simulink model "target_generation_test"  (R2016b)
settings: Solver=VariableStepAuto  StartTime=0.0  StopTime=1  RelTol=1e-3
values from neighbouring files (symbols this model uses):
  fsw_params = init_fsw_params()    [target_generation_test_init.m]
  sc2gs_eci_unit = [-0.2821; 0.7163; 0.6382]    [target_generation_test_init.m]
  sc2sun_eci_unit = zeros(3,1)    [target_generation_test_init.m]
  sc_mode = 31    [target_generation_test_init.m]
  sc_quat = [1; 0; 0; 0]    [target_generation_test_init.m]
  vel_eci_kmps = [0.9082; 0.3185; 0.2715]    [target_generation_test_init.m]
libraries: aerolibtransform2 x1, target_generation_lib x1
settings Model: Creator=Taylor  LastModifiedBy=taylorreynolds

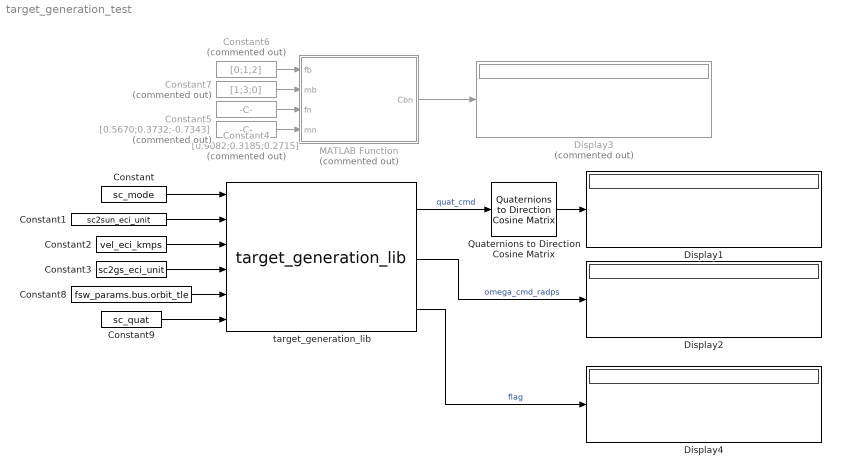
== system target_generation_test ==
  Constant : Constant  Value=sc_mode
  Constant1 : Constant  Value=sc2sun_eci_unit
  Constant2 : Constant  Value=vel_eci_kmps
  Constant3 : Constant  Value=sc2gs_eci_unit
  Constant4 : Constant  Commented=on  Value=[0.9082;0.3185;0.2715]
  Constant5 : Constant  Commented=on  Value=[0.5670;0.3732;-0.7343]
  Constant6 : Constant  Commented=on  Value=[0;1;2]
  Constant7 : Constant  Commented=on  Value=[1;3;0]
  Constant8 : Constant  Value=fsw_params.bus.orbit_tle
  Constant9 : Constant  Value=sc_quat
  Display1 : Display
  Display2 : Display
  Display3 : Display  Commented=on
  Display4 : Display
  MATLAB Function : MATLAB Function  Commented=on  TreatAsAtomicUnit=on
  Quaternions to Direction Cosine Matrix : aerolibtransform2/Quaternions to  Direction Cosine Matrix
  target_generation_lib : target_generation_lib/target_generation_lib
  wires:
  Constant/1 -> target_generation_lib/1
  Constant3/1 -> target_generation_lib/4
  Constant2/1 -> target_generation_lib/3
  Constant1/1 -> target_generation_lib/2
  target_generation_lib/1 -> Quaternions to Direction Cosine Matrix/1  "quat_cmd"
  Quaternions to Direction Cosine Matrix/1 -> Display1/1
  MATLAB Function/1(Cbn) -> Display3/1
  Constant7/1 -> MATLAB Function/2(mb)
  Constant6/1 -> MATLAB Function/1(fb)
  Constant5/1 -> MATLAB Function/4(mn)
  Constant4/1 -> MATLAB Function/3(fn)
  target_generation_lib/2 -> Display2/1  "omega_cmd_radps"
  Constant8/1 -> target_generation_lib/5
  Constant9/1 -> target_generation_lib/6
  target_generation_lib/3 -> Display4/1  "flag"

== matlab function target_generation_test/MATLAB Function ==
  data: fb input; Cbn output; mb input; fn input; mn input
function Cbn = TRIAD(fb, mb, fn, mn)
% Cbn = TRIAD(fb, mb, fn, mn)
% Function implements  TRIAD algorithm using measurements
% from three-component accelerometer with orthogonal axes and vector
% magnetometer
%
%   Input arguments:
%   fb  - Acceleration vector in body frame [3x1]
%   mb  - Magnetic field vector in body frame [3x1]
%   fn  - Gravity vector in navigation frame [3x1]
%   mn  - Magetic field vector in navigation frame [3x1]
%
%   Output arguments:
%   Cbn - estimated Direction Cosines Matrix (DCM)

W1 = fb/norm(fb);
W2 = mb/norm(mb);

V1 = fn;
V2 = mn;

Ou1 = W1;
Ou2 = cross(W1,W2)/norm(cross(W1,W2));
Ou3 = cross(W1,cross(W1,W2))/norm(cross(W1,W2));

R1 = V1;
R2 = cross(V1,V2)/norm(cross(V1,V2));
R3 = cross(V1,cross(V1,V2))/norm(cross(V1,V2));

Mou = [Ou1, Ou2, Ou3];
Mr = [R1, R2, R3];

%TRIAD DCM
Cbn = Mr*Mou';

end
